simulink model "Updated_Interstellar_R2020a"  (R2020a)
settings: Solver=VariableStepAuto  StartTime=0.0  StopTime=10.0  RelTol=1e-3
values from neighbouring files (symbols this model uses):
  g = 9.81    [Workspace.mat]
  rho = 1.184    [Workspace.mat]
  sensorCalibrationData = [0.09 -0.06 -9.473 -0.0095 -0.0075 0.0015 101270.95 0]    [Workspace.mat]
  Sensors =     [Workspace.mat]
  States =     [Workspace.mat]
  takeOffDuration = 1    [Workspace.mat]
undefined symbols (not defined in the file or in its folder): gray, Rec, SDTV, sigbuilder_block, strel
libraries: simulink x6, plantLibrary x1, visionfilter x1, visionmorphops x1, visionanalysis x1, parrotlib x1, visionconversions x1, sensorsLibrary x1
settings Model: Creator=user  LastModifiedBy=user

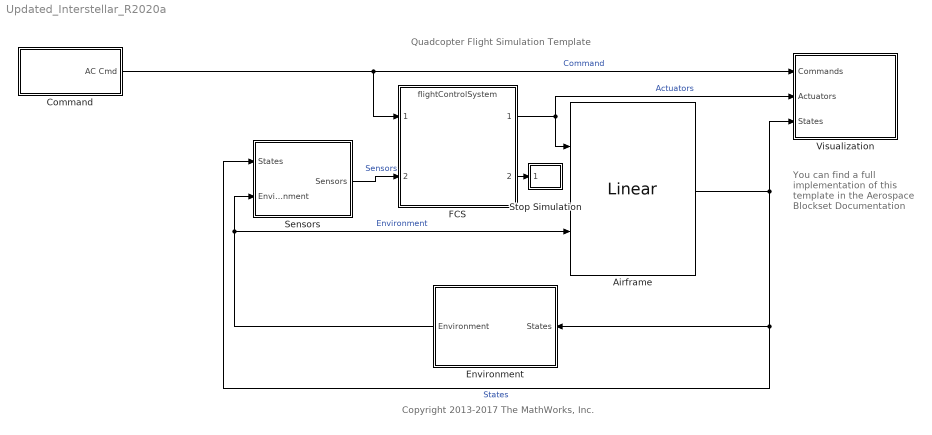
== system Updated_Interstellar_R2020a ==
  note: You can find a full implementation of this template in the
      | Aerospace Blockset Documentation
  note: Quadcopter Flight Simulation Template
  note: Copyright 2013-2017 The MathWorks, Inc.
  Airframe : plantLibrary/Linear  SystemSampleTime=-1  Latency=0  AutoFrameSizeCalculation=off
  Command : Subsystem  VariantControl=VSS_COMMAND_SIGBLDR
  Environment : Subsystem  TreatAsAtomicUnit=on  VariantControl=VSS_ENVIRONMENT_CST
  FCS : ModelReference  ModelNameDialog=flightControlSystem.slx  SimulationMode=Normal  ModelReferenceVersion=1.96
  Sensors : Subsystem  TreatAsAtomicUnit=on  VariantControl=VSS_SENSORS_FEEDTHROUGH
  Stop Simulation : Subsystem
  Visualization : Subsystem  VariantControl=VSS_VISUALIZATION_SCOPES
  wires:
  Sensors/1(Sensors) -> FCS/2  "Sensors"
  Environment/1(Environment) -> Airframe/2, Sensors/2(Environment)  "Environment"
  FCS/1 -> Airframe/1, Visualization/2(Actuators)  "Actuators"
  FCS/2 -> Stop Simulation/1(Flag)
  Airframe/1 -> Visualization/3(States), Environment/1(States), Sensors/1(States)  "States"
  Command/1(AC Cmd) -> Visualization/1(Commands), FCS/1  "Command"

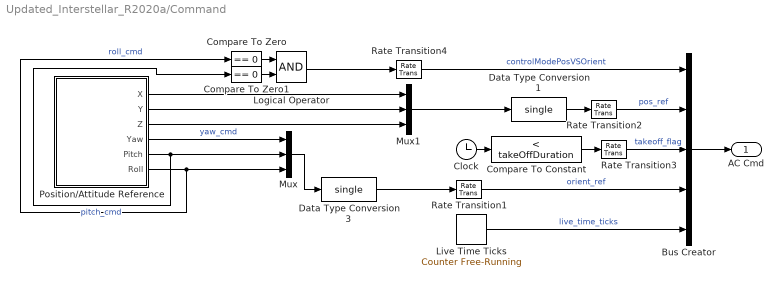
== system Updated_Interstellar_R2020a/Command ==
  Bus Creator : BusCreator  Inputs=5  OutDataTypeStr=Bus: CommandBus  NonVirtualBus=on
  Clock : Clock
  Compare To Constant : simulink/Logic and Bit Operations/Compare To Constant  relop=<  const=takeOffDuration  OutDataTypeStr=boolean
  Compare To Zero : simulink/Logic and Bit Operations/Compare To Zero  relop===  OutDataTypeStr=boolean
  Compare To Zero1 : simulink/Logic and Bit Operations/Compare To Zero  relop===  OutDataTypeStr=boolean
  Data Type Conversion1 : DataTypeConversion  OutDataTypeStr=single
  Data Type Conversion3 : DataTypeConversion  OutDataTypeStr=single
  Live Time Ticks : simulink/Sources/Counter Free-Running  NumBits=32  tsamp=Ts
  Logical Operator : Logic  AllPortsSameDT=off  OutDataTypeStr=boolean
  Mux : Mux  Inputs=3
  Mux1 : Mux  Inputs=3
  Position/Attitude Reference : Subsystem  Tag=STV Subsys  LoadFcn=sigbuilder_block('load');  StartFcn=sigbuilder_block('start');  StopFcn=sigbuilder_block('stop');  ClipboardFcn=sigbuilder_block('clipboard');  mask(Sigbuilder block){tuvar=[0:10]}
      mask help: Simulink:masks:SigbuilderBlock_MD
      mask init:
      | if ~strcmp(get_param(bdroot(gcbh),'SimulationStatus'),'stopped') tuvar = sigbuilder_block('maskInit'); end
      settings: CopyFcn=sigbuilder_block('copy');  DeleteFcn=sigbuilder_block('delete');  ModelCloseFcn=sigbuilder_block('modelClose');  PreSaveFcn=sigbuilder_block('preSave');  PauseFcn=sigbuilder_block('pause');  ContinueFcn=sigbuilder_block('continue');  NameChangeFcn=sigbuilder_block('namechange');  OpenFcn=sigbuilder_block('open',[435 197.25 555 408.75 ]);  CloseFcn=sigbuilder_block('close');
      mask Display: plot(0, 0, 100, 100,[2, 2, 32, 32, 2], [68, 8, 8, 68, 68],[32, 2], [38, 38], [32, 19, 2],[53, 60, 44], [32, 17, 17, 2],[16, 16, 31, 31]);txt = getActiveGroup(gcbh);text(2, 100, txt,'verticalAlignment', 'top');
  Rate Transition{1..4} (4 alike) : RateTransition  OutPortSampleTime=Ts
  AC Cmd : Outport  OutDataTypeStr=Bus: CommandBus  VectorParamsAs1DForOutWhenUnconnected=off
  wires:
  Bus Creator/1 -> AC Cmd/1
  Position/Attitude Reference/6(Roll) -> Compare To Zero/1, Mux/3  "roll_cmd"
  Position/Attitude Reference/5(Pitch) -> Mux/2, Compare To Zero1/1  "pitch_cmd"
  Position/Attitude Reference/4(Yaw) -> Mux/1  "yaw_cmd"
  Mux/1 -> Data Type Conversion3/1
  Data Type Conversion3/1 -> Rate Transition1/1
  Rate Transition1/1 -> Bus Creator/4  "orient_ref"
  Compare To Zero/1 -> Logical Operator/1
  Compare To Zero1/1 -> Logical Operator/2
  Logical Operator/1 -> Rate Transition4/1
  Rate Transition4/1 -> Bus Creator/1  "controlModePosVSOrient"
  Position/Attitude Reference/1(X) -> Mux1/1
  Position/Attitude Reference/2(Y) -> Mux1/2
  Position/Attitude Reference/3(Z) -> Mux1/3
  Mux1/1 -> Data Type Conversion1/1
  Data Type Conversion1/1 -> Rate Transition2/1
  Rate Transition2/1 -> Bus Creator/2  "pos_ref"
  Clock/1 -> Compare To Constant/1
  Compare To Constant/1 -> Rate Transition3/1
  Rate Transition3/1 -> Bus Creator/3  "takeoff_flag"
  Live Time Ticks/1 -> Bus Creator/5  "live_time_ticks"

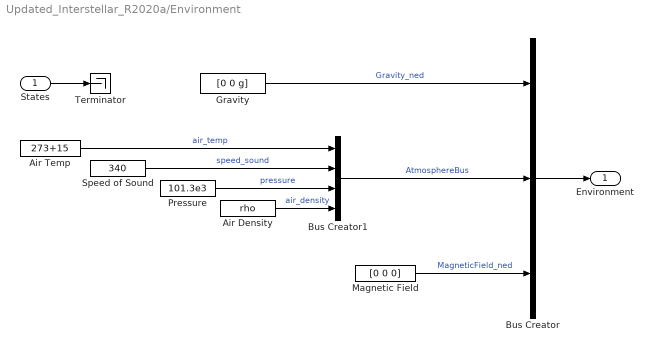
== system Updated_Interstellar_R2020a/Environment ==
  States : Inport  OutDataTypeStr=Bus: StatesBus
  Air Density : Constant  Value=rho
  Air Temp : Constant  Value=273+15
  Bus Creator : BusCreator  Inputs=3  OutDataTypeStr=Bus: EnvironmentBus  NonVirtualBus=on
  Bus Creator1 : BusCreator  Inputs=4  OutDataTypeStr=Bus: AtmosphereBus  NonVirtualBus=on
  Gravity : Constant  Value=[0 0 g]
  Magnetic Field : Constant  Value=[0 0 0]
  Pressure : Constant  Value=101.3e3
  Speed of Sound : Constant  Value=340
  Terminator : Terminator
  Environment : Outport  VectorParamsAs1DForOutWhenUnconnected=off
  wires:
  States/1 -> Terminator/1
  Gravity/1 -> Bus Creator/1  "Gravity_ned"
  Bus Creator/1 -> Environment/1
  Air Temp/1 -> Bus Creator1/1  "air_temp"
  Speed of Sound/1 -> Bus Creator1/2  "speed_sound"
  Pressure/1 -> Bus Creator1/3  "pressure"
  Air Density/1 -> Bus Creator1/4  "air_density"
  Bus Creator1/1 -> Bus Creator/2  "AtmosphereBus"
  Magnetic Field/1 -> Bus Creator/3  "MagneticField_ned"

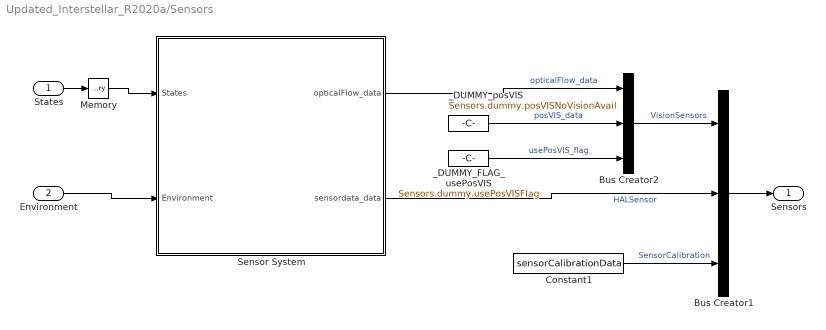
== system Updated_Interstellar_R2020a/Sensors ==
  States : Inport  OutDataTypeStr=Bus: StatesBus
  Environment : Inport  Port=2  OutDataTypeStr=Bus: EnvironmentBus
  Bus Creator1 : BusCreator  Inputs=3  OutDataTypeStr=Bus: SensorsBus  NonVirtualBus=on
  Bus Creator2 : BusCreator  Inputs=3  OutDataTypeStr=Bus: extraSensorData_t  NonVirtualBus=on
  Constant1 : Constant  Value=sensorCalibrationData  OutDataTypeStr=single
  Memory : Memory  InitialCondition=States  InheritSampleTime=on
  Sensor System : Subsystem
  _DUMMY_FLAG_usePosVIS : Constant  Value=Sensors.dummy.usePosVISFlag  OutDataTypeStr=single
  _DUMMY_posVIS : Constant  Value=Sensors.dummy.posVISNoVisionAvail  OutDataTypeStr=single
  Sensors : Outport  OutDataTypeStr=Bus: SensorsBus  VectorParamsAs1DForOutWhenUnconnected=off
  wires:
  Constant1/1 -> Bus Creator1/3  "SensorCalibration"
  Memory/1 -> Sensor System/1(States)
  Sensor System/2(sensordata_data) -> Bus Creator1/2  "HALSensor"
  States/1 -> Memory/1
  Environment/1 -> Sensor System/2(Environment)
  Bus Creator1/1 -> Sensors/1
  _DUMMY_FLAG_usePosVIS/1 -> Bus Creator2/3  "usePosVIS_flag"
  Sensor System/1(opticalFlow_data) -> Bus Creator2/1  "opticalFlow_data"
  _DUMMY_posVIS/1 -> Bus Creator2/2  "posVIS_data"
  Bus Creator2/1 -> Bus Creator1/1  "VisionSensors"

== system Updated_Interstellar_R2020a/Stop Simulation ==
  Flag : Inport
  Assertion : Assertion
  Compare To Zero : simulink/Logic and Bit Operations/Compare To Zero  relop=>  OutDataTypeStr=boolean
  Logical Operator : Logic  Operator=NOT  AllPortsSameDT=off  OutDataTypeStr=boolean
  wires:
  Flag/1 -> Compare To Zero/1
  Compare To Zero/1 -> Logical Operator/1
  Logical Operator/1 -> Assertion/1

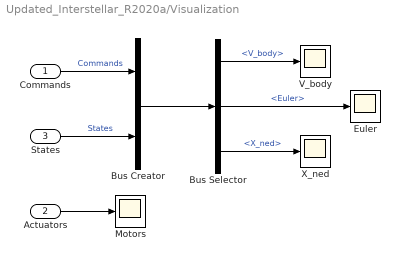
== system Updated_Interstellar_R2020a/Visualization ==
  Commands : Inport  OutDataTypeStr=Bus: CommandBus
  Actuators : Inport  Port=2
  States : Inport  Port=3  OutDataTypeStr=Bus: StatesBus
  Bus Creator : BusCreator  Inputs=2
  Bus Selector : BusSelector  OutputSignals=States.V_body,States.Euler,States.X_ned
  Euler : Scope
  Motors : Scope
  V_body : Scope
  X_ned : Scope
  wires:
  Commands/1 -> Bus Creator/1  "Commands"
  States/1 -> Bus Creator/2  "States"
  Bus Creator/1 -> Bus Selector/1
  Bus Selector/1 -> V_body/1  "<V_body>"
  Bus Selector/2 -> Euler/1  "<Euler>"
  Bus Selector/3 -> X_ned/1  "<X_ned>"
  Actuators/1 -> Motors/1

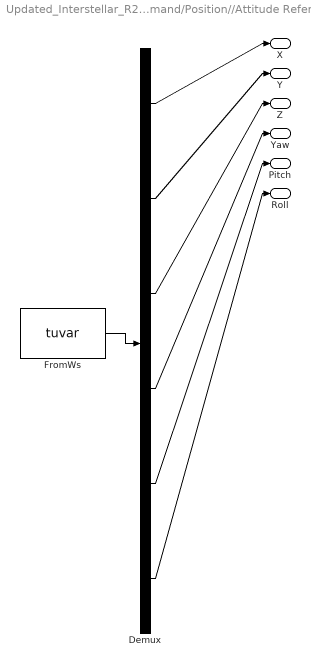
== system Updated_Interstellar_R2020a/Command/Position//Attitude Reference ==
  Demux : Demux  Tag=STV Demux  Outputs=6
      settings: DisplayOption=none
  FromWs : FromWorkspace  Tag=STV FromWs  VariableName=tuvar
      SigBuilderData=|
      | common.afterFinalStr = 'Extrapolate'
      | common.sampleTime = 0
      | dataSet.timeRange = [0 100]
      | dataSet.name = 'Group 1'
      | sbobj.Groups.Name = 'Group 1'
      | sbobj.Groups.Signals(1).Name = 'X'
      | sbobj.Groups.Signals(1).XData = [0 100]
      | sbobj.Groups.Signals(1).YData = [0 0]
      | sbobj.Groups.Signals(2).Name = 'Y'
      | sbobj.Groups.Signals(2).XData = [0 100]
      | sbobj.Groups.Signals(2).YData = [0 0]
      | sbobj.Groups.Signals(3).Name = 'Z'
      | sbobj.Groups.Signals(3).XData = [0 1 1 100]
      | sbobj.Groups.Signals(3).YData = [0 0 -1.5 -1.5]
      | sbobj.Groups.Signals(4).Name = 'Yaw'
      | sbobj.Groups.Signals(4).XData = [0 5.5 8 100]
      | sbobj.Groups.Signals(4).YData = [0 0 0 0]
      | sbobj.Groups.Signals(5).Name = 'Pitch'
      | sbobj.Groups.Signals(5).XData = [0 3 4 100]
      | sbobj.Groups.Signals(5).YData = [0 0 0 0]
      | sbobj.Groups.Signals(6).Name = 'Roll'
      | sbobj.Groups.Signals(6).XData = [0 100]
      | sbobj.Groups.Signals(6).YData = [0 0]
      | sbobj.Groups.TimeRange = [0 100]
  X : Outport  Tag=STV Outport  VectorParamsAs1DForOutWhenUnconnected=off
  Y : Outport  Tag=STV Outport  Port=2  VectorParamsAs1DForOutWhenUnconnected=off
  Z : Outport  Tag=STV Outport  Port=3  VectorParamsAs1DForOutWhenUnconnected=off
  Yaw : Outport  Tag=STV Outport  Port=4  VectorParamsAs1DForOutWhenUnconnected=off
  Pitch : Outport  Tag=STV Outport  Port=5  VectorParamsAs1DForOutWhenUnconnected=off
  Roll : Outport  Tag=STV Outport  Port=6  VectorParamsAs1DForOutWhenUnconnected=off
  wires:
  FromWs/1 -> Demux/1
  Demux/1 -> X/1
  Demux/2 -> Y/1
  Demux/3 -> Z/1
  Demux/4 -> Yaw/1
  Demux/5 -> Pitch/1
  Demux/6 -> Roll/1

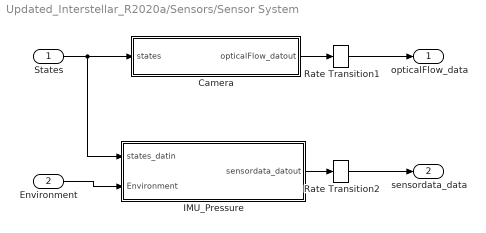
== system Updated_Interstellar_R2020a/Sensors/Sensor System ==
  States : Inport
  Environment : Inport  Port=2
  Camera : Subsystem  AncestorBlock=sensorsLibrary/Camera
  IMU_Pressure : Subsystem
  Rate Transition1 : RateTransition  OutPortSampleTime=Ts
  Rate Transition2 : RateTransition  OutPortSampleTime=Ts
  opticalFlow_data : Outport  VectorParamsAs1DForOutWhenUnconnected=off
  sensordata_data : Outport  Port=2  OutDataTypeStr=Bus: HAL_acquisition_t  VectorParamsAs1DForOutWhenUnconnected=off
  wires:
  Environment/1 -> IMU_Pressure/2(Environment)
  Camera/1(opticalFlow_datout) -> Rate Transition1/1
  IMU_Pressure/1(sensordata_datout) -> Rate Transition2/1
  Rate Transition1/1 -> opticalFlow_data/1
  Rate Transition2/1 -> sensordata_data/1
  States/1 -> Camera/1(states), IMU_Pressure/1(states_datin)

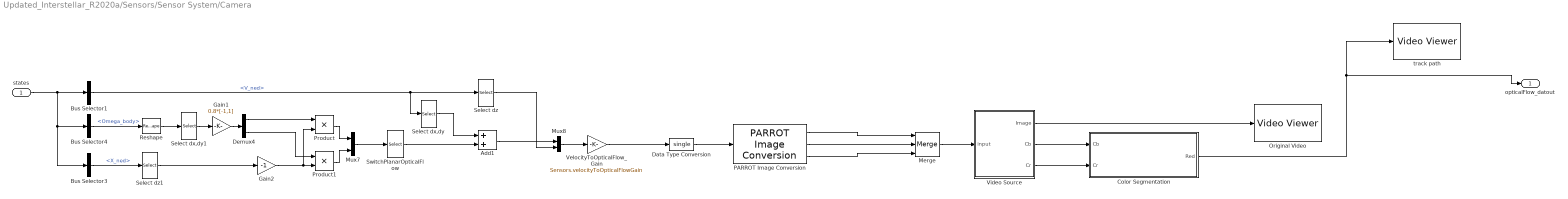
== system Updated_Interstellar_R2020a/Sensors/Sensor System/Camera ==
  states : Inport
  Add1 : Sum
  Bus Selector1 : BusSelector  OutputSignals=V_ned
  Bus Selector3 : BusSelector  OutputSignals=X_ned
  Bus Selector4 : BusSelector  OutputSignals=Omega_body
  Color Segmentation : Subsystem
  Data Type Conversion : DataTypeConversion  OutDataTypeStr=single
  Demux4 : Demux  Outputs=2
  Gain1 : Gain  Gain=0.8*[-1,1]
  Gain2 : Gain  Gain=-1
  Merge : Merge  Inputs=3
  Mux7 : Mux  Inputs=2
  Mux8 : Mux  Inputs=2
  Original Video : VideoViewer  colormapValue=gray(256)  FigPos=[685 765 681 682]  trueSizedOnce=on
  PARROT Image Conversion : parrotlib/PARROT Image Conversion  Tag=IP_FORMAT  ImageFormat=RGB  R=on  Y=on  G=on  U=on  B=on  V=on
  Product : Product
  Product1 : Product
  Reshape : Reshape
  Select dx,dy : Selector  InputPortWidth=3  IndexOptions=Index vector (dialog)  Indices=[1 2]  OutputSizes=1
  Select dx,dy1 : Selector  InputPortWidth=3  IndexOptions=Index vector (dialog)  Indices=[1 2]  OutputSizes=1
  Select dz : Selector  InputPortWidth=3  IndexOptions=Index vector (dialog)  Indices=3  OutputSizes=1
  Select dz1 : Selector  InputPortWidth=3  IndexOptions=Index vector (dialog)  Indices=3  OutputSizes=1
  SwitchPlanarOpticalFlow : Selector  InputPortWidth=2  IndexOptions=Index vector (dialog)  Indices=[2 1]  OutputSizes=1
  VelocityToOpticalFlow_Gain : Gain  Gain=Sensors.velocityToOpticalFlowGain
  "Video Source " : Subsystem
  "track path " : VideoViewer  colormapValue=gray(256)  FigPos=[1 766 683 691]  trueSizedOnce=on
  opticalFlow_datout : Outport  VectorParamsAs1DForOutWhenUnconnected=off
  wires:
  Reshape/1 -> Select dx,dy1/1
  Select dz1/1 -> Gain2/1
  VelocityToOpticalFlow_Gain/1 -> Data Type Conversion/1
  Mux8/1 -> VelocityToOpticalFlow_Gain/1
  Bus Selector4/1 -> Reshape/1  "<Omega_body>"
  Bus Selector3/1 -> Select dz1/1  "<X_ned>"
  Select dz/1 -> Mux8/2
  Add1/1 -> Mux8/1
  SwitchPlanarOpticalFlow/1 -> Add1/2
  Select dx,dy/1 -> Add1/1
  Gain2/1 -> Product1/2, Product/2
  Select dx,dy1/1 -> Gain1/1
  Mux7/1 -> SwitchPlanarOpticalFlow/1
  Product1/1 -> Mux7/2
  Product/1 -> Mux7/1
  Demux4/2 -> Product1/1
  Gain1/1 -> Demux4/1
  Demux4/1 -> Product/1
  Bus Selector1/1 -> Select dz/1, Select dx,dy/1  "<V_ned>"
  states/1 -> Bus Selector1/1, Bus Selector4/1, Bus Selector3/1
  "Video Source "/3(Cr) -> Color Segmentation/2(Cr)
  "Video Source "/2(Cb) -> Color Segmentation/1(Cb)
  "Video Source "/1(Image) -> Original Video/1
  Color Segmentation/1(Red) -> "track path "/1, opticalFlow_datout/1
  Data Type Conversion/1 -> PARROT Image Conversion/1
  Merge/1 -> "Video Source "/1("input ")
  PARROT Image Conversion/1 -> Merge/1
  PARROT Image Conversion/2 -> Merge/2
  PARROT Image Conversion/3 -> Merge/3

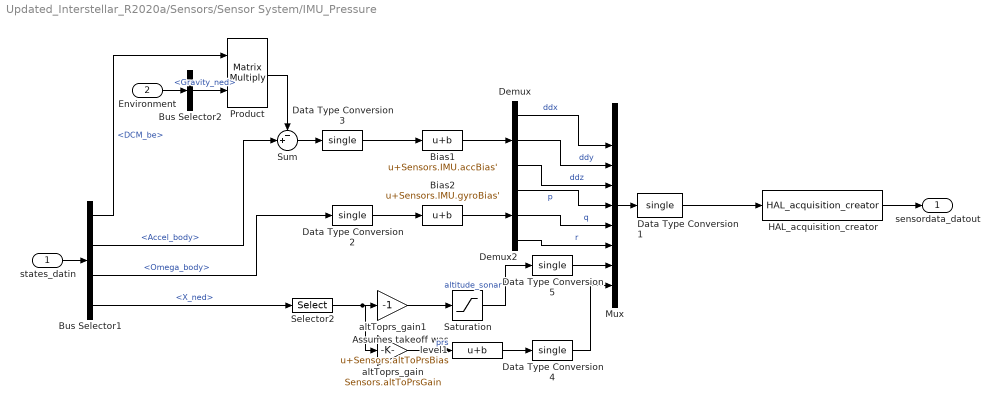
== system Updated_Interstellar_R2020a/Sensors/Sensor System/IMU_Pressure ==
  states_datin : Inport  OutDataTypeStr=Bus: StatesBus
  Environment : Inport  Port=2
  Assumes takeoff was level1 : Bias  Bias=Sensors.altToPrsBias
  Bias1 : Bias  Bias=Sensors.IMU.accBias'
  Bias2 : Bias  Bias=Sensors.IMU.gyroBias'
  Bus Selector1 : BusSelector  OutputSignals=DCM_be,Accel_body,Omega_body,X_ned
  Bus Selector2 : BusSelector  OutputSignals=Gravity_ned
  Data Type Conversion{1..5} (5 alike) : DataTypeConversion  OutDataTypeStr=single
  Demux : Demux  Outputs=3
  Demux2 : Demux  Outputs=3
  HAL_acquisition_creator : sensorsLibrary/HAL_acquisition_creator  SystemSampleTime=-1  Latency=0  AutoFrameSizeCalculation=off
  Mux : Mux  Inputs=9
  Product : Product  Multiplication=Matrix(*)
  Saturation : Saturate  UpperLimit=inf  LowerLimit=Sensors.altSensorMin  OutDataTypeStr=single
  Selector2 : Selector  InputPortWidth=3  IndexOptions=Index vector (dialog)  Indices=[3]  OutputSizes=1
  Sum : Sum  Inputs=-+|
  altToprs_gain : Gain  Gain=Sensors.altToPrsGain  ParamDataTypeStr=single  OutDataTypeStr=single
  altToprs_gain1 : Gain  Gain=-1  ParamDataTypeStr=single  OutDataTypeStr=single
  sensordata_datout : Outport  OutDataTypeStr=Bus: HAL_acquisition_t  VectorParamsAs1DForOutWhenUnconnected=off
  wires:
  Bias2/1 -> Demux2/1
  Bias1/1 -> Demux/1
  Product/1 -> Sum/1
  Bus Selector1/2 -> Sum/2  "<Accel_body>"
  Sum/1 -> Data Type Conversion3/1
  Bus Selector1/1 -> Product/1  "<DCM_be>"
  Bus Selector2/1 -> Product/2  "<Gravity_ned>"
  altToprs_gain1/1 -> Saturation/1
  Data Type Conversion5/1 -> Mux/8
  Data Type Conversion4/1 -> Mux/9
  Data Type Conversion2/1 -> Bias2/1
  Data Type Conversion3/1 -> Bias1/1
  Assumes takeoff was level1/1 -> Data Type Conversion4/1
  Bus Selector1/4 -> Selector2/1  "<X_ned>"
  states_datin/1 -> Bus Selector1/1
  Environment/1 -> Bus Selector2/1
  Bus Selector1/3 -> Data Type Conversion2/1  "<Omega_body>"
  HAL_acquisition_creator/1 -> sensordata_datout/1
  Data Type Conversion1/1 -> HAL_acquisition_creator/1
  Mux/1 -> Data Type Conversion1/1
  altToprs_gain/1 -> Assumes takeoff was level1/1  "prs"
  Saturation/1 -> Data Type Conversion5/1  "altitude_sonar"
  Selector2/1 -> altToprs_gain1/1, altToprs_gain/1
  Demux/3 -> Mux/4  "ddz"
  Demux2/3 -> Mux/7  "r"
  Demux/2 -> Mux/3  "ddy"
  Demux/1 -> Mux/2  "ddx"
  Demux2/1 -> Mux/5  "p"
  Demux2/2 -> Mux/6  "q"

== system Updated_Interstellar_R2020a/Sensors/Sensor System/Camera/Color Segmentation ==
  Cb : Inport
  Cr : Inport  Port=2
  Color Classifier : Subsystem
  Filtering : Subsystem
  Red : Outport
  wires:
  Color Classifier/1("Red ") -> Filtering/1(Red)
  Cb/1 -> Color Classifier/1(cb)
  Cr/1 -> Color Classifier/2(cr)
  Filtering/1(refined Red) -> Red/1

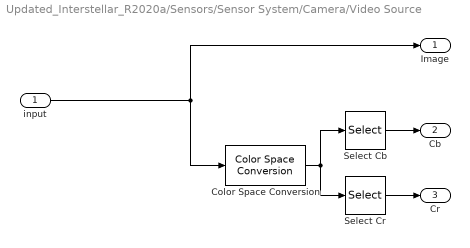
== system Updated_Interstellar_R2020a/Sensors/Sensor System/Camera/Video Source  ==
  "input " : Inport
  Color Space Conversion : visionconversions/Color Space  Conversion  conversion=Obsolete  conversionActive=R'G'B' to Y'CbCr  wp_str=D65  rec=Rec. 601 (SDTV)  sys=1125/60/2:1  imagePorts=One multidimensional signal
  Select Cb : Selector  NumberOfDimensions=3  InputPortWidth=3  IndexOptions=Select all,Select all,Index vector (dialog)  Indices=[1 3],1,2  OutputSizes=1,1,1
  Select Cr : Selector  NumberOfDimensions=3  InputPortWidth=3  IndexOptions=Select all,Select all,Index vector (dialog)  Indices=[1 3],1,3  OutputSizes=1,1,1
  Image : Outport
  Cb : Outport  Port=2
  Cr : Outport  Port=3
  wires:
  "input "/1 -> Color Space Conversion/1, Image/1
  Color Space Conversion/1 -> Select Cb/1, Select Cr/1
  Select Cb/1 -> Cb/1
  Select Cr/1 -> Cr/1

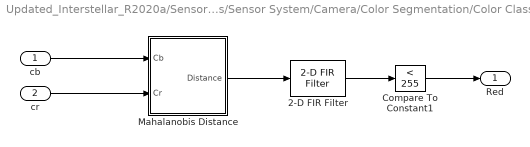
== system Updated_Interstellar_R2020a/Sensors/Sensor System/Camera/Color Segmentation/Color Classifier ==
  cb : Inport
  cr : Inport  Port=2
  2-D FIR Filter : visionfilter/2-D FIR Filter  separable=off  filtSrc=Specify via dialog  filterMtrx=single(1/9*ones(3))  verticalFilter=[4 0]  horizontalFilter=[4 0]  outSize=Full  padType=Constant  padSrc=Specify via dialog  padVal=0  method=Convolution  firstCoeffSignedness=Signed  firstCoeffLastDataTypeStr=Inherit: Same word length as input  outputMode=Binary point scaling  outputWordLength=32  outputFracLength=12  outputSignedness=Auto  outputLastDataTypeStr=fixdt([],32,12)  accumLastDataTypeStr=Inherit: Same as product output  prodOutputMode=Binary point scaling  prodOutputWordLength=32  prodOutputFracLength=10  prodOutputLastDataTypeStr=fixdt([],32,10)  roundingMode=Floor  overflowMode=off  firstCoeffDataTypeStr=Inherit: Same word length as input  firstCoeffMin=[]  firstCoeffMax=[]  prodOutputDataTypeStr=fixdt([],32,10)  accumDataTypeStr=Inherit: Same as product output  outputDataTypeStr=fixdt([],32,12)  outputMin=[]  outputMax=[]
      settings: SourceProductBaseCode=VP
  Compare To Constant1 : simulink/Logic and Bit Operations/Compare To Constant  relop=<  const=255  OutDataTypeStr=boolean  ZeroCross=off
  "Mahalanobis Distance " : Subsystem
  "Red " : Outport
  wires:
  "Mahalanobis Distance "/1(Distance) -> 2-D FIR Filter/1
  cb/1 -> "Mahalanobis Distance "/1(Cb)
  cr/1 -> "Mahalanobis Distance "/2(Cr)
  Compare To Constant1/1 -> "Red "/1
  2-D FIR Filter/1 -> Compare To Constant1/1

== system Updated_Interstellar_R2020a/Sensors/Sensor System/Camera/Color Segmentation/Filtering ==
  Red : Inport
  Closing : visionmorphops/Closing  nhoodsrc=Specify via dialog  strel=strel('disk',5)
      settings: SourceProductBaseCode=VP
  Median Filter : Subsystem
  refined Red : Outport
  wires:
  Red/1 -> Median Filter/1(Red)
  Median Filter/1(Filtered Red) -> Closing/1
  Closing/1 -> refined Red/1

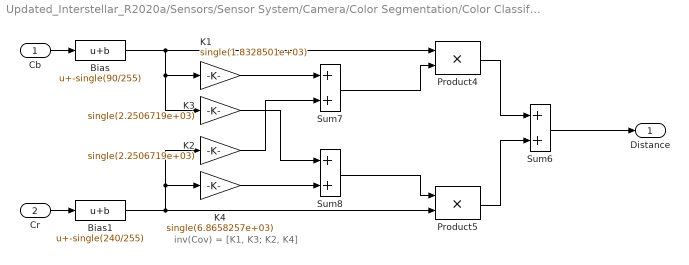
== system Updated_Interstellar_R2020a/Sensors/Sensor System/Camera/Color Segmentation/Color Classifier/Mahalanobis Distance  ==
  note: inv(Cov) = [K1, K3; K2, K4]
  Cb : Inport
  Cr : Inport  Port=2
  Bias : Bias  Bias=-single(90/255)
  Bias1 : Bias  Bias=-single(240/255)
  K1 : Gain  Gain=single(1.8328501e+03)  SaturateOnIntegerOverflow=on  OutDataTypeStr=Inherit: Same as input  ParamDataTypeStr=Inherit: Same as input
  K2 : Gain  Gain=single(2.2506719e+03)  SaturateOnIntegerOverflow=on  OutDataTypeStr=Inherit: Same as input  ParamDataTypeStr=Inherit: Same as input
  K3 : Gain  Gain=single(2.2506719e+03)  SaturateOnIntegerOverflow=on  OutDataTypeStr=Inherit: Same as input  ParamDataTypeStr=Inherit: Same as input
  K4 : Gain  Gain=single(6.8658257e+03)  SaturateOnIntegerOverflow=on  OutDataTypeStr=Inherit: Same as input  ParamDataTypeStr=Inherit: Same as input
  Product4 : Product  InputSameDT=on  SaturateOnIntegerOverflow=on  OutDataTypeStr=Inherit: Same as first input
  Product5 : Product  InputSameDT=on  SaturateOnIntegerOverflow=on  OutDataTypeStr=Inherit: Same as first input
  Sum6 : Sum  InputSameDT=on  SaturateOnIntegerOverflow=on  OutDataTypeStr=Inherit: Same as first input
  Sum7 : Sum  InputSameDT=on  SaturateOnIntegerOverflow=on  OutDataTypeStr=Inherit: Same as first input
  Sum8 : Sum  InputSameDT=on  SaturateOnIntegerOverflow=on  OutDataTypeStr=Inherit: Same as first input
  Distance : Outport
  wires:
  Cb/1 -> Bias/1
  Cr/1 -> Bias1/1
  K4/1 -> Sum8/2
  Product4/1 -> Sum6/1
  Product5/1 -> Sum6/2
  K1/1 -> Sum7/1
  K2/1 -> Sum7/2
  K3/1 -> Sum8/1
  Sum7/1 -> Product4/2
  Sum8/1 -> Product5/1
  Bias/1 -> Product4/1, K1/1, K3/1
  Bias1/1 -> Product5/2, K4/1, K2/1
  Sum6/1 -> Distance/1

== system Updated_Interstellar_R2020a/Sensors/Sensor System/Camera/Color Segmentation/Filtering/Median Filter ==
  Red : Inport
  Data Type Conversion5 : DataTypeConversion  OutDataTypeStr=boolean  SaturateOnIntegerOverflow=on  RndMeth=Zero
  Data Type Conversion6 : DataTypeConversion  OutDataTypeStr=single  SaturateOnIntegerOverflow=on  RndMeth=Zero
  Median Filter : visionanalysis/Median Filter  nghbood=[3 3]  outSize=Same as input port I  padType=Constant  padSrc=Specify via dialog  padVal=0  roundingMode=Floor  overflowMode=off
      settings: SourceProductBaseCode=VP
  Filtered Red : Outport
  wires:
  Red/1 -> Data Type Conversion6/1
  Data Type Conversion5/1 -> Filtered Red/1
  Median Filter/1 -> Data Type Conversion5/1
  Data Type Conversion6/1 -> Median Filter/1
